simulink model "WanderMultipleLM"  (R2019b)
settings: Solver=VariableStepAuto  StartTime=0.0  StopTime=30.0  RelTol=1e-3
values from neighbouring files (symbols this model uses):
  z = zeros(length(ofdx)*2+3*tracking_delay_length,1,length(out.ofd.time))    [panacea_1.m]    (also in panacea_2.m = zeros(length(ofdx)*2+3*tracking_delay_length+6,1); panacea_3.m = zeros(length(ofdx)*2+3*tracking_delay_length+6,1); panacea_4.m = zeros(length(ofdx)*2+3*tracking_delay_length+6,1); panacea_5.m = zeros(length(ofdx)*2+3*tracking_delay_length+6,1))
undefined symbols (not defined in the file or in its folder): f, globalTs, lms, numOfLm, phi, psi, the, x, y
libraries: simulink x7, sharedtransform x2
settings Model: Creator=thinhhoang  LastModifiedBy=thinhhoang

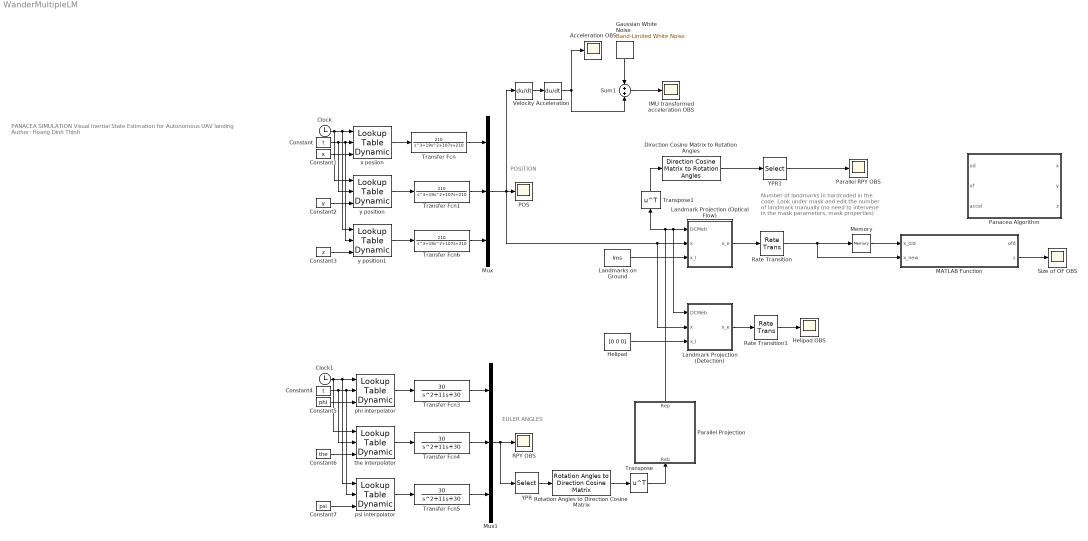
== system WanderMultipleLM ==
  note: PANACEA SIMULATION
      | Visual Inertial State Estimation for Autonomous UAV landing
      | Author: Hoang Dinh Thinh
  note: Number of landmarks in hardcoded in the code. Look under mask and edit the number of landmark manually (no need to intervene in the mask parameters, mask properties)
  note: POSITION
  note: EULER ANGLES
  Acceleration : Derivative
  Acceleration OBS : Scope
  Clock : Clock
  Clock1 : Clock
  Constant : Constant  Value=t
  Constant1 : Constant  Value=x
  Constant2 : Constant  Value=y
  Constant3 : Constant  Value=z
  Constant4 : Constant  Value=t
  Constant5 : Constant  Value=phi
  Constant6 : Constant  Value=the
  Constant7 : Constant  Value=psi
  Direction Cosine Matrix to Rotation Angles : sharedtransform/Direction Cosine Matrix to Rotation Angles  rotationOrder=ZYX  aMode=aMode  action=None  tolerance=eps(2)
      settings: SourceProductName=Aerospace Blockset  SourceProductBaseCode=AE
  Gaussian White Noise : simulink/Sources/Band-Limited White Noise  Cov=[1e-4]  Ts=globalTs  seed=[23341]
  Helipad : Constant  Value=[0 0 0]
  Helipad OBS : Scope
  IMU transformed acceleration OBS : Scope
  Landmark Projection (Detection) : MATLAB Function  TreatAsAtomicUnit=on  mask{f=f, numOfLm=1}
      mask prompts: f "Focal length"; numOfLm "Number of landmarks"
  Landmark Projection (Optical Flow) : MATLAB Function  TreatAsAtomicUnit=on  mask{f=f, numOfLm=numOfLm}
      mask prompts: f "Focal length"; numOfLm "Number of landmarks"
  Landmarks on Ground : Constant  Value=lms
  MATLAB Function : MATLAB Function  TreatAsAtomicUnit=on
  Memory : Memory
  Mux : Mux  Inputs=3
  Mux1 : Mux  Inputs=3
  POS : Scope
  Panacea Algorithm : MATLAB Function  TreatAsAtomicUnit=on
  Parallel Projection : MATLAB Function  TreatAsAtomicUnit=on
  Parallel RPY OBS : Scope
  RPY OBS : Scope
  Rate Transition : RateTransition  OutPortSampleTime=trackingTs
  Rate Transition1 : RateTransition  OutPortSampleTime=trackingTs
  Rotation Angles to Direction Cosine Matrix : sharedtransform/Rotation Angles to Direction Cosine Matrix  rotationOrder=ZYX  aMode=aMode
      settings: SourceProductBaseCode=AE
  Size of OF OBS : Scope
  Sum1 : Sum  Inputs=+|+
  Transfer Fcn : TransferFcn  Numerator=[210]  Denominator=[1 19 107 210]
  Transfer Fcn1 : TransferFcn  Numerator=[210]  Denominator=[1 19 107 210]
  Transfer Fcn3 : TransferFcn  Numerator=[30]  Denominator=[1 11 30]
  Transfer Fcn4 : TransferFcn  Numerator=[30]  Denominator=[1 11 30]
  Transfer Fcn5 : TransferFcn  Numerator=[30]  Denominator=[1 11 30]
  Transfer Fcn6 : TransferFcn  Numerator=[210]  Denominator=[1 19 107 210]
  Transpose : Math  Operator=transpose  SignedPower=off  SaturateOnIntegerOverflow=on
  Transpose1 : Math  Operator=transpose  SignedPower=off  SaturateOnIntegerOverflow=on
  Velocity : Derivative
  YPR : Selector  InputPortWidth=3  IndexOptions=Index vector (dialog)  Indices=[3 2 1]  OutputSizes=1
  YPR1 : Selector  InputPortWidth=3  IndexOptions=Index vector (dialog)  Indices=[3 2 1]  OutputSizes=1
  phi interpolator : simulink/Lookup Tables/Lookup Table Dynamic  LookUpMeth=Interpolation-Use End Values  OutDataType=fixdt('double')  OutScaling=[]  OutputDataTypeScalingMode=Specify via dialog  OutDataTypeStr=double  DoSatur=off
      settings: SourceProductName=Simulink
  psi interpolator : simulink/Lookup Tables/Lookup Table Dynamic  LookUpMeth=Interpolation-Use End Values  OutDataType=fixdt('double')  OutScaling=[]  OutputDataTypeScalingMode=Specify via dialog  OutDataTypeStr=double  DoSatur=off
      settings: SourceProductName=Simulink
  the interpolator : simulink/Lookup Tables/Lookup Table Dynamic  LookUpMeth=Interpolation-Use End Values  OutDataType=fixdt('double')  OutScaling=[]  OutputDataTypeScalingMode=Specify via dialog  OutDataTypeStr=double  DoSatur=off
      settings: SourceProductName=Simulink
  x posiion : simulink/Lookup Tables/Lookup Table Dynamic  LookUpMeth=Interpolation-Use End Values  OutDataType=fixdt('double')  OutScaling=[]  OutputDataTypeScalingMode=Specify via dialog  OutDataTypeStr=double  DoSatur=off
      settings: SourceProductName=Simulink
  y position : simulink/Lookup Tables/Lookup Table Dynamic  LookUpMeth=Interpolation-Use End Values  OutDataType=fixdt('double')  OutScaling=[]  OutputDataTypeScalingMode=Specify via dialog  OutDataTypeStr=double  DoSatur=off
      settings: SourceProductName=Simulink
  y position1 : simulink/Lookup Tables/Lookup Table Dynamic  LookUpMeth=Interpolation-Use End Values  OutDataType=fixdt('double')  OutScaling=[]  OutputDataTypeScalingMode=Specify via dialog  OutDataTypeStr=double  DoSatur=off
      settings: SourceProductName=Simulink
  wires:
  Clock/1 -> y position/1, y position1/1, x posiion/1
  Constant/1 -> y position/2, y position1/2, x posiion/2
  Constant1/1 -> x posiion/3
  Constant2/1 -> y position/3
  Constant3/1 -> y position1/3
  x posiion/1 -> Transfer Fcn/1
  Transfer Fcn/1 -> Mux/1
  Mux/1 -> Velocity/1, Landmark Projection (Detection)/2(x), Landmark Projection (Optical Flow)/2(x), POS/1
  Clock1/1 -> the interpolator/1, psi interpolator/1, phi interpolator/1
  Constant4/1 -> the interpolator/2, psi interpolator/2, phi interpolator/2
  Constant5/1 -> phi interpolator/3
  Constant6/1 -> the interpolator/3
  Constant7/1 -> psi interpolator/3
  phi interpolator/1 -> Transfer Fcn3/1
  the interpolator/1 -> Transfer Fcn4/1
  psi interpolator/1 -> Transfer Fcn5/1
  Transfer Fcn3/1 -> Mux1/1
  Transfer Fcn4/1 -> Mux1/2
  Transfer Fcn5/1 -> Mux1/3
  Mux1/1 -> YPR/1, RPY OBS/1
  YPR/1 -> Rotation Angles to Direction Cosine Matrix/1
  Rotation Angles to Direction Cosine Matrix/1 -> Transpose/1
  Landmarks on Ground/1 -> Landmark Projection (Optical Flow)/3(x_l)
  Transpose/1 -> Parallel Projection/1(Reb)
  Parallel Projection/1(Rep) -> Landmark Projection (Detection)/1(DCMeb), Landmark Projection (Optical Flow)/1(DCMeb), Transpose1/1
  Transpose1/1 -> Direction Cosine Matrix to Rotation Angles/1
  Direction Cosine Matrix to Rotation Angles/1 -> YPR1/1
  YPR1/1 -> Parallel RPY OBS/1
  Landmark Projection (Optical Flow)/1(x_e) -> Rate Transition/1
  Velocity/1 -> Acceleration/1
  Acceleration/1 -> Sum1/2, Acceleration OBS/1
  Transfer Fcn1/1 -> Mux/2
  y position/1 -> Transfer Fcn1/1
  y position1/1 -> Transfer Fcn6/1
  Transfer Fcn6/1 -> Mux/3
  Gaussian White Noise/1 -> Sum1/1
  Sum1/1 -> IMU transformed acceleration OBS/1
  Rate Transition/1 -> MATLAB Function/2(x_new), Memory/1
  Memory/1 -> MATLAB Function/1(x_old)
  MATLAB Function/2(s) -> Size of OF OBS/1
  Helipad/1 -> Landmark Projection (Detection)/3(x_l)
  Landmark Projection (Detection)/1(x_e) -> Rate Transition1/1
  Rate Transition1/1 -> Helipad OBS/1

== matlab function WanderMultipleLM/Parallel Projection ==
  data: Reb input; Rep output
function Rep = ParallelProjection(Reb)
Rpb = ParallelProject(Reb);
Rep = Rpb'*Reb;
end

== matlab function WanderMultipleLM/Landmark Projection (Optical Flow) ==
  data: DCMeb input size=[3 3]; x input size=[1 3]; x_l input size=[numOfLm 3]; x_e output size=[numOfLm 2]; f parameter size=1; numOfLm parameter size=1
function x_e  = pi(DCMeb, x, x_l, f, numOfLm)
    x_e = zeros(50, 2);
    for i=1:numOfLm
        x_e(i,:) = Project(f, DCMeb, x, x_l(i,:));
    end
end

== matlab function WanderMultipleLM/MATLAB Function ==
  data: x_old input; ofd output; x_new input; s output size=1
function [ofd, s] = OpticalFlowEstimator(x_old, x_new)
    numOfLm = length(x_old);
    ofd = zeros(numOfLm, 2);
    k = 0;
    for i=1:numOfLm
        if (x_old(i,1)==-1 || x_old(i,2)==-1 || x_new(i,1)==-1 || x_new(i,2)==-1)
            ofd(i,:) = [0 0];
        else
            ofd(i,:) = x_new(i,:) - x_old(i,:);
            k = k+1;
        end
    end
    s = k;
end

== matlab function WanderMultipleLM/Panacea Algorithm ==
  data: x output; od input; y output; of input; accel input; z output
function [x,y,z]= PanaceaAlg(od, of, accel)

y = u;

== matlab function WanderMultipleLM/Landmark Projection (Detection) ==
  data: DCMeb input size=[3 3]; x input size=[1 3]; x_l input size=[numOfLm 3]; x_e output size=[numOfLm 2]; f parameter size=1; numOfLm parameter size=1
function x_e  = pi(DCMeb, x, x_l, f, numOfLm)
    x_e = zeros(1, 2);
    for i=1:numOfLm
        x_e(i,:) = Project(f, DCMeb, x, x_l(i,:));
    end
end
